simulink model "System_Design_Quadrocopter"  (Simulink 7.5)
settings: Solver=ode45  StartTime=0.0  StopTime=30  RelTol=1e-3
values from neighbouring files (symbols this model uses):
  phi0 = 0.15    [Quadrocopter_control_Driver.m]    (also in calc_stability.m = 0)
  r_phi0 = 0    [Quadrocopter_control_Driver.m]    (also in calc_stability.m)
  r_psi0 = 0    [Quadrocopter_control_Driver.m]    (also in calc_stability.m)
  r_theta0 = 0    [Quadrocopter_control_Driver.m]    (also in calc_stability.m)
  theta0 = 0.15    [Quadrocopter_control_Driver.m]    (also in calc_stability.m = 0)
  Ts = 0.01    [Reglerauslegung.m]    (also in Test_Reglerauslegung.m)
undefined symbols (not defined in the file or in its folder): bodyCtrl_phiCtrl_KD, bodyCtrl_phiCtrl_KI, bodyCtrl_phiCtrl_KP, bodyCtrl_rphiCtrl_KD, bodyCtrl_rphiCtrl_KI, bodyCtrl_rphiCtrl_KP, bodyCtrl_rpsiCtrl_KD, bodyCtrl_rpsiCtrl_KI, bodyCtrl_rpsiCtrl_KP, bodyCtrl_rthetaCtrl_KD, bodyCtrl_rthetaCtrl_KI, bodyCtrl_rthetaCtrl_KP, bodyCtrl_thetaCtrl_KD, bodyCtrl_thetaCtrl_KI, bodyCtrl_thetaCtrl_KP, boom, f1, f2, f3, f4, f5, g, I_x, I_y, I_z, m, positionCtrl_rpsiCtrl_KD, positionCtrl_rpsiCtrl_KI, positionCtrl_rpsiCtrl_KP, sigbuilder_block, speed, thrust, Ts_Opt
libraries: simulink x39, dspobslib x4, Copter_Library x3, Control_lib x1, sdolib x1
(part 3 of 4)

== system System_Design_Quadrocopter/Quadrocopter/Remote Control/Remote_Control_3d_mouse ==
  note: phi(roll)
      | theta(pitch)
      | rpsi(yaw rate)
      | T(thrust)
  Enable : EnablePort  PropagateVarSize=During execution
  Add : Sum
  Add1 : Sum
  Add2 : Sum
  Constant1 : Constant  Value=128
  Constant2 : Constant  Value=128
  Constant3 : Constant  Value=400
  Constant4 : Constant  Value=128
  Demux : Demux  Outputs=3
  Demux1 : Demux  Outputs=3
  Gain1 : Gain
  Mux2 : Mux
  Saturation : Saturate  UpperLimit=255  LowerLimit=0
  Saturation1 : Saturate  UpperLimit=255  LowerLimit=0
  Saturation2 : Saturate  UpperLimit=255  LowerLimit=0
  Saturation3 : Saturate  UpperLimit=inf  LowerLimit=0
  Space Mouse Input : S-Function  AncestorBlock=vrlib/Space Mouse Input  FunctionName=spacemouse  Parameters=Port, OutputType, InitialPosition, InitialRotation, PositionSensitivity, RotationSensitivity, Dominant, NormalizeAngle, DisableTranslation, DisableRotation, PositionLow, PositionUp, EnableLimit  EnableBusSupport=off  mask(Space Mouse Input){Port=USB1, OutputType=Speed, Dominant=off, DisableTranslation=off, DisableRotation=off, NormalizeAngle=off, EnableLimit=on, PositionSensitivity=0.5, RotationSensitivity=2, InitialPosition=[0 0 0], InitialRotation=[0 0 0], PositionLow=[0 0 0], PositionUp=[255 255 255]}
      mask prompts: OutputType "Output type:"; Dominant "Dominant mode"; DisableTranslation "Disable position movement"; DisableRotation "Disable rotation movement"; NormalizeAngle "Normalize output angle"; EnableLimit "Limit position"; PositionSensitivity "Position sensitivity:"; RotationSensitivity "Rotation sensitivity:"; InitialPosition "Initial position:"; InitialRotation "Initial rotation:"; PositionLow "Lower position limit:"; PositionUp "Upper position limit:"
      mask help: Space Mouse input device driver.
      mask Help: helpview(fullfile(docroot, 'toolbox', 'sl3d', 'sl3d.map'), 'vr_magellanspacemouse');
      mask StyleString: popup(COM1|COM2|COM3|COM4|USB1|USB2|USB3|USB4|USB),popup(Speed|Position|Viewpoint coordinates),checkbox,checkbox,checkbox,checkbox,checkbox,edit,edit,edit,edit,edit,edit
      mask CallbackString: spacemousemask|spacemousemask|||||spacemousemask||||||
      mask Display:
      | image(imread('spacemouseicon.png'))
      | port_label('output', 1, 'Translation')
      | port_label('output', 2, 'Rotation')
      | port_label('output', 3, 'Buttons')
  Out1 : Outport
  wires:
  Demux/1 -> Add2/1  "phi_set"
  Constant4/1 -> Add2/2
  Demux/3 -> Add1/1  "theta_set"
  Constant2/1 -> Add1/2
  Add/1 -> Saturation2/1
  Demux1/2 -> Add/1  "psi_set"
  Constant1/1 -> Add/2
  Space Mouse Input/2 -> Demux1/1  "[Kippen, Rollen, Drehen]"
  Space Mouse Input/1 -> Demux/1  "[Trans_X, Trans_Z, Trans_Y]"
  Gain1/1 -> Mux2/4  "thrust"
  Mux2/1 -> Out1/1
  Add2/1 -> Saturation/1
  Add1/1 -> Saturation1/1
  Saturation1/1 -> Mux2/2
  Saturation2/1 -> Mux2/3
  Saturation/1 -> Mux2/1
  Saturation3/1 -> Gain1/1
  Demux/2 -> Saturation3/1  "Zoom"

== system System_Design_Quadrocopter/Quadrocopter/Remote Control/Square_path_stimuli ==
  note: phi(roll)
      | theta(pitch)
      | rpsi(yaw rate)
      | T(thrust)
  Add{,1..3} (4 alike) : Sum  OutDataType=fixdt(1, 16)  OutScaling=2^-10
  Constant{,1..3} (4 alike) : Constant  Value=128  OutDataType=fixdt(1, 16)  OutScaling=2^0
  Gain : Gain  ParameterDataType=fixdt(1, 16)  ParameterScaling=2^0  OutDataType=fixdt(1, 16)  OutScaling=2^0
  Mux1 : Mux
  Signal Builder : Subsystem  Tag=STV Subsys  LoadFcn=sigbuilder_block('load');  StartFcn=sigbuilder_block('start');  StopFcn=sigbuilder_block('stop');  ClipboardFcn=sigbuilder_block('clipboard');  mask(Sigbuilder block){}
      mask help: Create and generate interchangeable groups of signals whose waveforms are piecewise linear.
      mask init:
      | if ~strcmp(get_param(bdroot(gcbh),'SimulationStatus'),'stopped') tuvar = sigbuilder_block('maskInit'); end
      settings: CopyFcn=sigbuilder_block('copy');  DeleteFcn=sigbuilder_block('delete');  ModelCloseFcn=sigbuilder_block('modelClose');  PreSaveFcn=sigbuilder_block('preSave');  NameChangeFcn=sigbuilder_block('namechange');  OpenFcn=sigbuilder_block('open',[437.25 199.5 550.5 399.75 ]);  CloseFcn=sigbuilder_block('close');
      mask Display: plot(0,0,100,100,[10,10,40,40,10],[80,20,20,80,80],[40,10],[50,50], [40,27,10],[65,72,56],[40,25,25,10],[28,28,43,43]);
  Subsystem1 : Subsystem  mask{Gain_=-40}
      mask prompts: Gain_ "Gain"
  Subsystem2 : Subsystem  mask{Gain_=-40}
      mask prompts: Gain_ "Gain"
  Subsystem3 : Subsystem  mask{Gain_=40}
      mask prompts: Gain_ "Gain"
  Subsystem4 : Subsystem  mask{Gain_=40}
      mask prompts: Gain_ "Gain"
  Out : Outport  OutDataType=fixdt(1, 16)  OutScaling=2^0
  wires:
  Mux1/1 -> Out/1
  Constant2/1 -> Mux1/3  "rpsi_set"
  Constant/1 -> Gain/1
  Gain/1 -> Mux1/4  "thrust"
  Subsystem3/1(Out1) -> Add1/1
  Subsystem1/1(Out1) -> Add1/2
  Constant3/1 -> Add/1
  Add/1 -> Mux1/1
  Subsystem4/1(Out1) -> Add2/1
  Subsystem2/1(Out1) -> Add2/2
  Add2/1 -> Add/2
  Add1/1 -> Add3/2
  Add3/1 -> Mux1/2
  Constant1/1 -> Add3/1
  Signal Builder/1(Signal 1) -> Subsystem4/1(In1)
  Signal Builder/2(Signal 2) -> Subsystem3/1(In1)
  Signal Builder/3(Signal 3) -> Subsystem2/1(In1)
  Signal Builder/4(Signal 4) -> Subsystem1/1(In1)

== system System_Design_Quadrocopter/Quadrocopter/Remote Control/Step_Stimuli ==
  note: phi(roll)
      | theta(pitch)
      | rpsi(yaw rate)
      | T(thrust)
  Add : Sum  OutDataType=fixdt(1, 16)  OutScaling=2^-10
  Add1 : Sum  OutDataType=fixdt(1, 16)  OutScaling=2^-10
  Add2 : Sum  OutDataType=fixdt(1, 16)  OutScaling=2^-10
  Constant{,1,3..4} (4 alike) : Constant  Value=128  OutDataType=fixdt(1, 16)  OutScaling=2^0
  Gain : Gain  ParameterDataType=fixdt(1, 16)  ParameterScaling=2^0  OutDataType=fixdt(1, 16)  OutScaling=2^0
  Mux1 : Mux
  Step_phi : Step  Time=[5]  After=[-128]  SampleTime=0
  Step_psi : Step  Time=[0]  After=[0]  SampleTime=0
  Step_theta : Step  Time=[5]  After=[0]  SampleTime=0
  Out : Outport  OutDataType=fixdt(1, 16)  OutScaling=2^0
  wires:
  Mux1/1 -> Out/1
  Constant/1 -> Gain/1
  Gain/1 -> Mux1/4  "thrust"
  Constant3/1 -> Add/2
  Add/1 -> Mux1/1
  Step_theta/1 -> Add1/1
  Constant4/1 -> Add1/2
  Add1/1 -> Mux1/2
  Step_psi/1 -> Add2/1
  Constant1/1 -> Add2/2
  Add2/1 -> Mux1/3
  Step_phi/1 -> Add/1

== system System_Design_Quadrocopter/Quadrocopter/SDO/captrPsi ==
  In2 : Inport
  Terminator : Terminator
  To File : ToFile  Filename=SDO_51.mat
  cntr : Constant  Value=<binary blob, 1398102 chars, not shown>  OutDataType=fixdt(1, 16)  OutScaling=2^0
  wires:
  In2/1 -> To File/1
  cntr/1 -> Terminator/1

== system System_Design_Quadrocopter/Quadrocopter/Sensors/Optical System ==
  note: %opt_sensor_record
      | %[
      | 1:Opt_Var_Trans
      | 2:Opt_Var_ST_Trans
      | 3:Opt_Limit_Trans
      | 4:Opt_Ori_SG_Trans
      | 5:Opt_Var_Rot
      | 6:Opt_Var_ST_Rot
      | 7:Opt_Limit_Rot
      | 8:Opt_Ori_SG_Rot
      | 9:Opt_Delay_Global
      | 10:Opt_ST_Global]
  IdealSigs : Inport
  Demux1 : Demux  Outputs=3
  Mux1 : Mux  Inputs=3
  Rotation rpsi : Subsystem  mask{Opt_Var=Opt_Sens_Rec(5), Opt_Var_ST=Opt_Sens_Rec(6), Opt_Limit=Opt_Sens_Rec(7), Opt_Delay=Opt_Sens_Rec(9), Opt_ST=Opt_Sens_Rec(10), Opt_Ori_SG=Opt_Sens_Rec(8)}
      mask prompts: Opt_Var "Variance"; Opt_Var_ST "Sample Time of Variance"; Opt_Limit "Limitation [m/s]"; Opt_Delay "Delay"; Opt_ST "Sample Time (1/Frame Rate)"; Opt_Ori_SG "Original Signal Gain"
  Scope : Scope
      settings: YMin=-0.5  YMax=7  SaveName=ScopeData23
  Translation VX : Subsystem  mask{Opt_Var=Opt_Sens_Rec(1), Opt_Var_ST=Opt_Sens_Rec(2), Opt_Limit=Opt_Sens_Rec(3), Opt_Delay=Opt_Sens_Rec(9), Opt_ST=Opt_Sens_Rec(10), Opt_Ori_SG=Opt_Sens_Rec(4)}
      mask prompts: Opt_Var "Variance"; Opt_Var_ST "Sample Time of Variance"; Opt_Limit "Limitation [m/s]"; Opt_Delay "Delay"; Opt_ST "Sample Time (1/Frame Rate)"; Opt_Ori_SG "Original Signal Gain"
  Translation VY : Subsystem  mask{Opt_Var=Opt_Sens_Rec(1), Opt_Var_ST=Opt_Sens_Rec(2), Opt_Limit=Opt_Sens_Rec(3), Opt_Delay=Opt_Sens_Rec(9), Opt_ST=Opt_Sens_Rec(10), Opt_Ori_SG=Opt_Sens_Rec(4)}
      mask prompts: Opt_Var "Variance"; Opt_Var_ST "Sample Time of Variance"; Opt_Limit "Limitation [m/s]"; Opt_Delay "Delay"; Opt_ST "Sample Time (1/Frame Rate)"; Opt_Ori_SG "Original Signal Gain"
  SensorSigs : Outport
  wires:
  Demux1/1 -> Translation VX/1(IdealSig)
  Demux1/2 -> Translation VY/1(IdealSig)
  Demux1/3 -> Rotation rpsi/1(IdealSig)
  Translation VX/1(OptSig) -> Mux1/1
  Translation VY/1(OptSig) -> Mux1/2
  Rotation rpsi/1(OptSig) -> Mux1/3
  IdealSigs/1 -> Demux1/1
  Mux1/1 -> SensorSigs/1, Scope/1

== system System_Design_Quadrocopter/Quadrocopter/Sensors/acc_ax_sensor ==
  note: inverted work like the real copter
  ax : Inport
  Enable Noise : Inport  Port=2
  Gain17 : Gain  Gain=g
  Gain30 : Gain  Gain=-340/g
  Quantizer4 : Quantizer  QuantizationInterval=g/340  SampleTime=Ts
  Saturation : Saturate  UpperLimit=6*g  LowerLimit=-6*g  OutDataType=fixdt(1, 16)  OutScaling=2^0
  Sensor Noise : Subsystem
  Sum15 : Sum
  Trigonometric Function : Trigonometry
  ax_sens : Outport
  wires:
  Sensor Noise/1(Noise) -> Sum15/1
  Sum15/1 -> Saturation/1
  Gain17/1 -> Sum15/2
  Quantizer4/1 -> Gain30/1
  Gain30/1 -> ax_sens/1
  Enable Noise/1 -> Sensor Noise/Enable
  Saturation/1 -> Quantizer4/1
  ax/1 -> Trigonometric Function/1
  Trigonometric Function/1 -> Gain17/1

== system System_Design_Quadrocopter/Quadrocopter/Sensors/acc_ay_sensor ==
  note: inverted like in the real copter
  phi : Inport
  Enable Noise : Inport  Port=2
  Gain19 : Gain  Gain=-340/g
  Gain22 : Gain  Gain=g
  Quantizer3 : Quantizer  QuantizationInterval=g/340  SampleTime=Ts
  Saturation : Saturate  UpperLimit=6*g  LowerLimit=-6*g  OutDataType=fixdt(1, 16)  OutScaling=2^0
  Sensor Noise : Subsystem
  Sum12 : Sum
  Trigonometric Function : Trigonometry
  ay_sens : Outport
  wires:
  Sum12/1 -> Saturation/1
  Quantizer3/1 -> Gain19/1
  phi/1 -> Trigonometric Function/1
  Gain19/1 -> ay_sens/1
  Enable Noise/1 -> Sensor Noise/Enable
  Sensor Noise/1(Noise) -> Sum12/1
  Saturation/1 -> Quantizer3/1
  Gain22/1 -> Sum12/2
  Trigonometric Function/1 -> Gain22/1

== system System_Design_Quadrocopter/Quadrocopter/Sensors/rate_phi_sensor ==
  note: Sensor adds noise and Samples and quantize the Signal. In combination with the gain a integer value is generated
      | like the Sensor is read from the ADC registers.
  r_phi : Inport
  Enable Noise : Inport  Port=2
  Gain20 : Gain  Gain=1/0.00938349
  Offset : Constant  Value=505
  Quantizer : Quantizer  QuantizationInterval=0.00938349  SampleTime=Ts
  Sensor Noise : Subsystem
  Sum : Sum  Inputs=++|
  Sum14 : Sum
  r_phi_sens : Outport
  wires:
  Sum14/1 -> Quantizer/1
  Quantizer/1 -> Gain20/1
  r_phi/1 -> Sum14/2
  Gain20/1 -> Sum/2
  Offset/1 -> Sum/1
  Sum/1 -> r_phi_sens/1
  Enable Noise/1 -> Sensor Noise/Enable
  Sensor Noise/1(Noise) -> Sum14/1

== system System_Design_Quadrocopter/Quadrocopter/Sensors/rate_psi_sensor ==
  note: Gyroscope / Acceleration Sensor
  sig_in : Inport
  enable_noise_in : Inport  Port=2
  Gain : Gain  Gain=-1/0.00938349
  Offset : Constant  Value=505
  Quantizer : Quantizer  QuantizationInterval=0.00938349  SampleTime=Ts
  Sensor Noise : Subsystem
  Sum : Sum  Inputs=++|
  Sum13 : Sum
  sens_out : Outport
  wires:
  Sensor Noise/1(Noise) -> Sum13/1
  sig_in/1 -> Sum13/2
  Offset/1 -> Sum/1
  Gain/1 -> Sum/2
  Sum/1 -> sens_out/1
  enable_noise_in/1 -> Sensor Noise/Enable
  Quantizer/1 -> Gain/1
  Sum13/1 -> Quantizer/1

== system System_Design_Quadrocopter/Quadrocopter/Sensors/rate_theta_sensor ==
  note: inverted to worj like in the real copter
  r_theta : Inport
  Enable Noise : Inport  Port=2
  Gain27 : Gain  Gain=-1/0.00938349
  Offset : Constant  Value=505
  Quantizer1 : Quantizer  QuantizationInterval=0.00938349  SampleTime=Ts
  Sensor Noise : Subsystem
  Sum : Sum  Inputs=++|
  Sum16 : Sum
  r_theta_sens : Outport
  wires:
  Sum16/1 -> Quantizer1/1
  Quantizer1/1 -> Gain27/1
  r_theta/1 -> Sum16/2
  Offset/1 -> Sum/1
  Gain27/1 -> Sum/2
  Sum/1 -> r_theta_sens/1
  Enable Noise/1 -> Sensor Noise/Enable
  Sensor Noise/1(Noise) -> Sum16/1

== system System_Design_Quadrocopter/Quadrocopter/Control/PID_Control_IMU Rot Trans (OC)/Control Hovering Mode ==
  vx_opt : Inport  OutDataType=fixdt(1, 16)  OutScaling=2^0
  theta_hm_set : Inport  Port=2  OutDataType=fixdt(1, 16)  OutScaling=2^0
  phi_hm_set : Inport  Port=3  OutDataType=fixdt(1, 16)  OutScaling=2^0
  vy_opt : Inport  Port=4  OutDataType=fixdt(1, 16)  OutScaling=2^0
  rpsi_opt : Inport  Port=5  OutDataType=fixdt(1, 16)  OutScaling=2^0
  rpsi_hm_set : Inport  Port=6  OutDataType=fixdt(1, 16)  OutScaling=2^0
  Enable : EnablePort  ZeroCross=off
  Gain : Gain  ParameterDataType=fixdt(1, 16)  ParameterScaling=2^0  OutDataType=fixdt(1, 16)  OutScaling=2^0
  Gain1 : Gain  ParameterDataType=fixdt(1, 16)  ParameterScaling=2^0  OutDataType=fixdt(1, 16)  OutScaling=2^0
  Gain6 : Gain  ParameterDataType=fixdt(1, 16)  ParameterScaling=2^0  OutDataType=fixdt(1, 16)  OutScaling=2^0
  PID rPhi OPT : simulink/Continuous/PID Controller  DialogController=pidpack.PIDConfig.pidDDGCreate  DialogControllerArgs=DataTag6  SystemSampleTime=-1  Controller=PID  TimeDomain=Discrete-time  SampleTime=Ts_Opt  IntegratorMethod=Forward Euler  FilterMethod=Forward Euler  Form=Ideal  P=10  I=0.5  D=0  N=2  InitialConditionSource=internal  InitialConditionForIntegrator=0  InitialConditionForFilter=0  ExternalReset=none  ZeroCross=off  LimitOutput=off  UpperSaturationLimit=inf  LowerSaturationLimit=-inf  LinearizeAsGain=off  AntiWindupMode=clamping  Kb=1  TrackingMode=off  Kt=1  PParamMin=[]  PParamMax=[]  IParamMin=[]  IParamMax=[]  DParamMin=[]  DParamMax=[]  NParamMin=[]  NParamMax=[]  KbParamMin=[]  KbParamMax=[]  KtParamMin=[]  KtParamMax=[]  POutMin=[]  POutMax=[]  IOutMin=[]  IOutMax=[]  DOutMin=[]  DOutMax=[]  NOutMin=[]  NOutMax=[]  KbOutMin=[]  KbOutMax=[]  KtOutMin=[]  KtOutMax=[]  IntegratorOutMin=[]  IntegratorOutMax=[]  FilterOutMin=[]  FilterOutMax=[]  SumOutMin=[]  SumOutMax=[]  SumI1OutMin=[]  SumI1OutMax=[]  SumI2OutMin=[]  SumI2OutMax=[]  SumI3OutMin=[]  SumI3OutMax=[]  SumDOutMin=[]  SumDOutMax=[]  SaturationOutMin=[]  SaturationOutMax=[]  IntegratorContinuousStateAttributes=''  IntegratorStateMustResolveToSignalObject=off  IntegratorRTWStateStorageClass=Auto  FilterContinuousStateAttributes=''  FilterStateMustResolveToSignalObject=off  FilterRTWStateStorageClass=Auto
  PID rPsi OPT : simulink/Continuous/PID Controller  DialogController=pidpack.PIDConfig.pidDDGCreate  DialogControllerArgs=DataTag7  SystemSampleTime=-1  Controller=PID  TimeDomain=Discrete-time  SampleTime=Ts_Opt  IntegratorMethod=Forward Euler  FilterMethod=Forward Euler  Form=Ideal  P=10  I=0.5  D=0  N=0  InitialConditionSource=internal  InitialConditionForIntegrator=0  InitialConditionForFilter=0  ExternalReset=none  ZeroCross=off  LimitOutput=off  UpperSaturationLimit=inf  LowerSaturationLimit=-inf  LinearizeAsGain=off  AntiWindupMode=clamping  Kb=1  TrackingMode=off  Kt=1  PParamMin=[]  PParamMax=[]  IParamMin=[]  IParamMax=[]  DParamMin=[]  DParamMax=[]  NParamMin=[]  NParamMax=[]  KbParamMin=[]  KbParamMax=[]  KtParamMin=[]  KtParamMax=[]  POutMin=[]  POutMax=[]  IOutMin=[]  IOutMax=[]  DOutMin=[]  DOutMax=[]  NOutMin=[]  NOutMax=[]  KbOutMin=[]  KbOutMax=[]  KtOutMin=[]  KtOutMax=[]  IntegratorOutMin=[]  IntegratorOutMax=[]  FilterOutMin=[]  FilterOutMax=[]  SumOutMin=[]  SumOutMax=[]  SumI1OutMin=[]  SumI1OutMax=[]  SumI2OutMin=[]  SumI2OutMax=[]  SumI3OutMin=[]  SumI3OutMax=[]  SumDOutMin=[]  SumDOutMax=[]  SaturationOutMin=[]  SaturationOutMax=[]  IntegratorContinuousStateAttributes=''  IntegratorStateMustResolveToSignalObject=off  IntegratorRTWStateStorageClass=Auto  FilterContinuousStateAttributes=''  FilterStateMustResolveToSignalObject=off  FilterRTWStateStorageClass=Auto
  PID rTheta OPT : simulink/Continuous/PID Controller  DialogController=pidpack.PIDConfig.pidDDGCreate  DialogControllerArgs=DataTag8  SystemSampleTime=-1  Controller=PID  TimeDomain=Discrete-time  SampleTime=Ts_Opt  IntegratorMethod=Forward Euler  FilterMethod=Forward Euler  Form=Ideal  P=10  I=0.5  D=0  N=0  InitialConditionSource=internal  InitialConditionForIntegrator=0  InitialConditionForFilter=0  ExternalReset=none  ZeroCross=off  LimitOutput=off  UpperSaturationLimit=inf  LowerSaturationLimit=-inf  LinearizeAsGain=off  AntiWindupMode=clamping  Kb=1  TrackingMode=off  Kt=1  PParamMin=[]  PParamMax=[]  IParamMin=[]  IParamMax=[]  DParamMin=[]  DParamMax=[]  NParamMin=[]  NParamMax=[]  KbParamMin=[]  KbParamMax=[]  KtParamMin=[]  KtParamMax=[]  POutMin=[]  POutMax=[]  IOutMin=[]  IOutMax=[]  DOutMin=[]  DOutMax=[]  NOutMin=[]  NOutMax=[]  KbOutMin=[]  KbOutMax=[]  KtOutMin=[]  KtOutMax=[]  IntegratorOutMin=[]  IntegratorOutMax=[]  FilterOutMin=[]  FilterOutMax=[]  SumOutMin=[]  SumOutMax=[]  SumI1OutMin=[]  SumI1OutMax=[]  SumI2OutMin=[]  SumI2OutMax=[]  SumI3OutMin=[]  SumI3OutMax=[]  SumDOutMin=[]  SumDOutMax=[]  SaturationOutMin=[]  SaturationOutMax=[]  IntegratorContinuousStateAttributes=''  IntegratorStateMustResolveToSignalObject=off  IntegratorRTWStateStorageClass=Auto  FilterContinuousStateAttributes=''  FilterStateMustResolveToSignalObject=off  FilterRTWStateStorageClass=Auto
  Sum1 : Sum  Inputs=|+-  OutDataType=fixdt(1, 16)  OutScaling=2^0
  Sum16 : Sum  Inputs=|+-  OutDataType=fixdt(1, 16)  OutScaling=2^0
  Sum2 : Sum  Inputs=|+-  OutDataType=fixdt(1, 16)  OutScaling=2^0
  m_theta : Outport  OutDataType=fixdt(1, 16)  OutScaling=2^0
  m_phi : Outport  Port=2  OutDataType=fixdt(1, 16)  OutScaling=2^0
  m_psi : Outport  Port=3  OutDataType=fixdt(1, 16)  OutScaling=2^0
  wires:
  Gain6/1 -> Sum16/2
  Sum16/1 -> PID rTheta OPT/1  "e_theta_hm"
  theta_hm_set/1 -> Sum16/1
  Sum2/1 -> PID rPhi OPT/1  "e_phi_hm"
  PID rPhi OPT/1 -> m_phi/1
  Gain1/1 -> Sum2/2
  vx_opt/1 -> Gain6/1
  PID rTheta OPT/1 -> m_theta/1
  phi_hm_set/1 -> Sum2/1
  rpsi_hm_set/1 -> Sum1/1
  PID rPsi OPT/1 -> Gain/1
  vy_opt/1 -> Gain1/1
  Sum1/1 -> PID rPsi OPT/1
  rpsi_opt/1 -> Sum1/2
  Gain/1 -> m_psi/1

== system System_Design_Quadrocopter/Quadrocopter/Control/PID_Control_IMU Rot Trans (OC) EMP/Control Hovering Mode ==
  vx_opt : Inport  OutDataType=fixdt(1, 16)  OutScaling=2^0
  theta_hm_set : Inport  Port=2  OutDataType=fixdt(1, 16)  OutScaling=2^0
  phi_hm_set : Inport  Port=3  OutDataType=fixdt(1, 16)  OutScaling=2^0
  vy_opt : Inport  Port=4  OutDataType=fixdt(1, 16)  OutScaling=2^0
  rpsi_opt : Inport  Port=5  OutDataType=fixdt(1, 16)  OutScaling=2^0
  rpsi_hm_set : Inport  Port=6  OutDataType=fixdt(1, 16)  OutScaling=2^0
  Enable : EnablePort  ZeroCross=off
  Gain : Gain  ParameterDataType=fixdt(1, 16)  ParameterScaling=2^0  OutDataType=fixdt(1, 16)  OutScaling=2^0
  Gain1 : Gain  ParameterDataType=fixdt(1, 16)  ParameterScaling=2^0  OutDataType=fixdt(1, 16)  OutScaling=2^0
  Gain6 : Gain  ParameterDataType=fixdt(1, 16)  ParameterScaling=2^0  OutDataType=fixdt(1, 16)  OutScaling=2^0
  PID rPhi OPT : simulink/Continuous/PID Controller  DialogController=pidpack.PIDConfig.pidDDGCreate  DialogControllerArgs=DataTag14  SystemSampleTime=-1  Controller=PID  TimeDomain=Discrete-time  SampleTime=Ts_Opt  IntegratorMethod=Forward Euler  FilterMethod=Forward Euler  Form=Ideal  P=10  I=0.5  D=0  N=2  InitialConditionSource=internal  InitialConditionForIntegrator=0  InitialConditionForFilter=0  ExternalReset=none  ZeroCross=off  LimitOutput=off  UpperSaturationLimit=inf  LowerSaturationLimit=-inf  LinearizeAsGain=off  AntiWindupMode=clamping  Kb=1  TrackingMode=off  Kt=1  PParamMin=[]  PParamMax=[]  IParamMin=[]  IParamMax=[]  DParamMin=[]  DParamMax=[]  NParamMin=[]  NParamMax=[]  KbParamMin=[]  KbParamMax=[]  KtParamMin=[]  KtParamMax=[]  POutMin=[]  POutMax=[]  IOutMin=[]  IOutMax=[]  DOutMin=[]  DOutMax=[]  NOutMin=[]  NOutMax=[]  KbOutMin=[]  KbOutMax=[]  KtOutMin=[]  KtOutMax=[]  IntegratorOutMin=[]  IntegratorOutMax=[]  FilterOutMin=[]  FilterOutMax=[]  SumOutMin=[]  SumOutMax=[]  SumI1OutMin=[]  SumI1OutMax=[]  SumI2OutMin=[]  SumI2OutMax=[]  SumI3OutMin=[]  SumI3OutMax=[]  SumDOutMin=[]  SumDOutMax=[]  SaturationOutMin=[]  SaturationOutMax=[]  IntegratorContinuousStateAttributes=''  IntegratorStateMustResolveToSignalObject=off  IntegratorRTWStateStorageClass=Auto  FilterContinuousStateAttributes=''  FilterStateMustResolveToSignalObject=off  FilterRTWStateStorageClass=Auto
  PID rPsi OPT : simulink/Continuous/PID Controller  DialogController=pidpack.PIDConfig.pidDDGCreate  DialogControllerArgs=DataTag15  SystemSampleTime=-1  Controller=PID  TimeDomain=Discrete-time  SampleTime=Ts_Opt  IntegratorMethod=Forward Euler  FilterMethod=Forward Euler  Form=Ideal  P=positionCtrl_rpsiCtrl_KP  I=positionCtrl_rpsiCtrl_KI  D=positionCtrl_rpsiCtrl_KD  N=0  InitialConditionSource=internal  InitialConditionForIntegrator=0  InitialConditionForFilter=0  ExternalReset=none  ZeroCross=off  LimitOutput=off  UpperSaturationLimit=inf  LowerSaturationLimit=-inf  LinearizeAsGain=off  AntiWindupMode=clamping  Kb=1  TrackingMode=off  Kt=1  PParamMin=[]  PParamMax=[]  IParamMin=[]  IParamMax=[]  DParamMin=[]  DParamMax=[]  NParamMin=[]  NParamMax=[]  KbParamMin=[]  KbParamMax=[]  KtParamMin=[]  KtParamMax=[]  POutMin=[]  POutMax=[]  IOutMin=[]  IOutMax=[]  DOutMin=[]  DOutMax=[]  NOutMin=[]  NOutMax=[]  KbOutMin=[]  KbOutMax=[]  KtOutMin=[]  KtOutMax=[]  IntegratorOutMin=[]  IntegratorOutMax=[]  FilterOutMin=[]  FilterOutMax=[]  SumOutMin=[]  SumOutMax=[]  SumI1OutMin=[]  SumI1OutMax=[]  SumI2OutMin=[]  SumI2OutMax=[]  SumI3OutMin=[]  SumI3OutMax=[]  SumDOutMin=[]  SumDOutMax=[]  SaturationOutMin=[]  SaturationOutMax=[]  IntegratorContinuousStateAttributes=''  IntegratorStateMustResolveToSignalObject=off  IntegratorRTWStateStorageClass=Auto  FilterContinuousStateAttributes=''  FilterStateMustResolveToSignalObject=off  FilterRTWStateStorageClass=Auto
  PID rTheta OPT : simulink/Continuous/PID Controller  DialogController=pidpack.PIDConfig.pidDDGCreate  DialogControllerArgs=DataTag16  SystemSampleTime=-1  Controller=PID  TimeDomain=Discrete-time  SampleTime=Ts_Opt  IntegratorMethod=Forward Euler  FilterMethod=Forward Euler  Form=Ideal  P=10  I=0.5  D=0  N=0  InitialConditionSource=internal  InitialConditionForIntegrator=0  InitialConditionForFilter=0  ExternalReset=none  ZeroCross=off  LimitOutput=off  UpperSaturationLimit=inf  LowerSaturationLimit=-inf  LinearizeAsGain=off  AntiWindupMode=clamping  Kb=1  TrackingMode=off  Kt=1  PParamMin=[]  PParamMax=[]  IParamMin=[]  IParamMax=[]  DParamMin=[]  DParamMax=[]  NParamMin=[]  NParamMax=[]  KbParamMin=[]  KbParamMax=[]  KtParamMin=[]  KtParamMax=[]  POutMin=[]  POutMax=[]  IOutMin=[]  IOutMax=[]  DOutMin=[]  DOutMax=[]  NOutMin=[]  NOutMax=[]  KbOutMin=[]  KbOutMax=[]  KtOutMin=[]  KtOutMax=[]  IntegratorOutMin=[]  IntegratorOutMax=[]  FilterOutMin=[]  FilterOutMax=[]  SumOutMin=[]  SumOutMax=[]  SumI1OutMin=[]  SumI1OutMax=[]  SumI2OutMin=[]  SumI2OutMax=[]  SumI3OutMin=[]  SumI3OutMax=[]  SumDOutMin=[]  SumDOutMax=[]  SaturationOutMin=[]  SaturationOutMax=[]  IntegratorContinuousStateAttributes=''  IntegratorStateMustResolveToSignalObject=off  IntegratorRTWStateStorageClass=Auto  FilterContinuousStateAttributes=''  FilterStateMustResolveToSignalObject=off  FilterRTWStateStorageClass=Auto
  Sum1 : Sum  Inputs=|+-  OutDataType=fixdt(1, 16)  OutScaling=2^0
  Sum16 : Sum  Inputs=|+-  OutDataType=fixdt(1, 16)  OutScaling=2^0
  Sum2 : Sum  Inputs=|+-  OutDataType=fixdt(1, 16)  OutScaling=2^0
  m_theta : Outport  OutDataType=fixdt(1, 16)  OutScaling=2^0
  m_phi : Outport  Port=2  OutDataType=fixdt(1, 16)  OutScaling=2^0
  m_psi : Outport  Port=3  OutDataType=fixdt(1, 16)  OutScaling=2^0
  wires:
  Gain6/1 -> Sum16/2
  Sum16/1 -> PID rTheta OPT/1  "e_theta_hm"
  theta_hm_set/1 -> Sum16/1
  Sum2/1 -> PID rPhi OPT/1  "e_phi_hm"
  PID rPhi OPT/1 -> m_phi/1
  Gain1/1 -> Sum2/2
  vx_opt/1 -> Gain6/1
  PID rTheta OPT/1 -> m_theta/1
  phi_hm_set/1 -> Sum2/1
  rpsi_hm_set/1 -> Sum1/1
  PID rPsi OPT/1 -> Gain/1
  vy_opt/1 -> Gain1/1
  Sum1/1 -> PID rPsi OPT/1
  rpsi_opt/1 -> Sum1/2
  Gain/1 -> m_psi/1

== system System_Design_Quadrocopter/Quadrocopter/Control/PID_Control_IMU only Trans (OC)/Control Hovering Mode ==
  vx_opt : Inport  OutDataType=fixdt(1, 16)  OutScaling=2^0
  theta_hm_set : Inport  Port=2  OutDataType=fixdt(1, 16)  OutScaling=2^0
  phi_hm_set : Inport  Port=3  OutDataType=fixdt(1, 16)  OutScaling=2^0
  vy_opt : Inport  Port=4  OutDataType=fixdt(1, 16)  OutScaling=2^0
  rpsi_opt : Inport  Port=5  OutDataType=fixdt(1, 16)  OutScaling=2^0
  rpsi_hm_set : Inport  Port=6  OutDataType=fixdt(1, 16)  OutScaling=2^0
  Enable : EnablePort  ZeroCross=off
  Gain : Gain  ParameterDataType=fixdt(1, 16)  ParameterScaling=2^0  OutDataType=fixdt(1, 16)  OutScaling=2^0
  Gain1 : Gain  ParameterDataType=fixdt(1, 16)  ParameterScaling=2^0  OutDataType=fixdt(1, 16)  OutScaling=2^0
  Gain6 : Gain  ParameterDataType=fixdt(1, 16)  ParameterScaling=2^0  OutDataType=fixdt(1, 16)  OutScaling=2^0
  PID rPhi OPT : simulink/Continuous/PID Controller  DialogController=pidpack.PIDConfig.pidDDGCreate  DialogControllerArgs=DataTag22  SystemSampleTime=-1  Controller=PID  TimeDomain=Discrete-time  SampleTime=Ts_Opt  IntegratorMethod=Forward Euler  FilterMethod=Forward Euler  Form=Ideal  P=10  I=0.5  D=0  N=2  InitialConditionSource=internal  InitialConditionForIntegrator=0  InitialConditionForFilter=0  ExternalReset=none  ZeroCross=off  LimitOutput=off  UpperSaturationLimit=inf  LowerSaturationLimit=-inf  LinearizeAsGain=off  AntiWindupMode=clamping  Kb=1  TrackingMode=off  Kt=1  PParamMin=[]  PParamMax=[]  IParamMin=[]  IParamMax=[]  DParamMin=[]  DParamMax=[]  NParamMin=[]  NParamMax=[]  KbParamMin=[]  KbParamMax=[]  KtParamMin=[]  KtParamMax=[]  POutMin=[]  POutMax=[]  IOutMin=[]  IOutMax=[]  DOutMin=[]  DOutMax=[]  NOutMin=[]  NOutMax=[]  KbOutMin=[]  KbOutMax=[]  KtOutMin=[]  KtOutMax=[]  IntegratorOutMin=[]  IntegratorOutMax=[]  FilterOutMin=[]  FilterOutMax=[]  SumOutMin=[]  SumOutMax=[]  SumI1OutMin=[]  SumI1OutMax=[]  SumI2OutMin=[]  SumI2OutMax=[]  SumI3OutMin=[]  SumI3OutMax=[]  SumDOutMin=[]  SumDOutMax=[]  SaturationOutMin=[]  SaturationOutMax=[]  IntegratorContinuousStateAttributes=''  IntegratorStateMustResolveToSignalObject=off  IntegratorRTWStateStorageClass=Auto  FilterContinuousStateAttributes=''  FilterStateMustResolveToSignalObject=off  FilterRTWStateStorageClass=Auto
  PID rPsi OPT : simulink/Continuous/PID Controller  DialogController=pidpack.PIDConfig.pidDDGCreate  DialogControllerArgs=DataTag23  SystemSampleTime=-1  Controller=PID  TimeDomain=Discrete-time  SampleTime=Ts_Opt  IntegratorMethod=Forward Euler  FilterMethod=Forward Euler  Form=Ideal  P=10  I=0.5  D=0  N=0  InitialConditionSource=internal  InitialConditionForIntegrator=0  InitialConditionForFilter=0  ExternalReset=none  ZeroCross=off  LimitOutput=off  UpperSaturationLimit=inf  LowerSaturationLimit=-inf  LinearizeAsGain=off  AntiWindupMode=clamping  Kb=1  TrackingMode=off  Kt=1  PParamMin=[]  PParamMax=[]  IParamMin=[]  IParamMax=[]  DParamMin=[]  DParamMax=[]  NParamMin=[]  NParamMax=[]  KbParamMin=[]  KbParamMax=[]  KtParamMin=[]  KtParamMax=[]  POutMin=[]  POutMax=[]  IOutMin=[]  IOutMax=[]  DOutMin=[]  DOutMax=[]  NOutMin=[]  NOutMax=[]  KbOutMin=[]  KbOutMax=[]  KtOutMin=[]  KtOutMax=[]  IntegratorOutMin=[]  IntegratorOutMax=[]  FilterOutMin=[]  FilterOutMax=[]  SumOutMin=[]  SumOutMax=[]  SumI1OutMin=[]  SumI1OutMax=[]  SumI2OutMin=[]  SumI2OutMax=[]  SumI3OutMin=[]  SumI3OutMax=[]  SumDOutMin=[]  SumDOutMax=[]  SaturationOutMin=[]  SaturationOutMax=[]  IntegratorContinuousStateAttributes=''  IntegratorStateMustResolveToSignalObject=off  IntegratorRTWStateStorageClass=Auto  FilterContinuousStateAttributes=''  FilterStateMustResolveToSignalObject=off  FilterRTWStateStorageClass=Auto
  PID rTheta OPT : simulink/Continuous/PID Controller  DialogController=pidpack.PIDConfig.pidDDGCreate  DialogControllerArgs=DataTag24  SystemSampleTime=-1  Controller=PID  TimeDomain=Discrete-time  SampleTime=Ts_Opt  IntegratorMethod=Forward Euler  FilterMethod=Forward Euler  Form=Ideal  P=10  I=0.5  D=0  N=0  InitialConditionSource=internal  InitialConditionForIntegrator=0  InitialConditionForFilter=0  ExternalReset=none  ZeroCross=off  LimitOutput=off  UpperSaturationLimit=inf  LowerSaturationLimit=-inf  LinearizeAsGain=off  AntiWindupMode=clamping  Kb=1  TrackingMode=off  Kt=1  PParamMin=[]  PParamMax=[]  IParamMin=[]  IParamMax=[]  DParamMin=[]  DParamMax=[]  NParamMin=[]  NParamMax=[]  KbParamMin=[]  KbParamMax=[]  KtParamMin=[]  KtParamMax=[]  POutMin=[]  POutMax=[]  IOutMin=[]  IOutMax=[]  DOutMin=[]  DOutMax=[]  NOutMin=[]  NOutMax=[]  KbOutMin=[]  KbOutMax=[]  KtOutMin=[]  KtOutMax=[]  IntegratorOutMin=[]  IntegratorOutMax=[]  FilterOutMin=[]  FilterOutMax=[]  SumOutMin=[]  SumOutMax=[]  SumI1OutMin=[]  SumI1OutMax=[]  SumI2OutMin=[]  SumI2OutMax=[]  SumI3OutMin=[]  SumI3OutMax=[]  SumDOutMin=[]  SumDOutMax=[]  SaturationOutMin=[]  SaturationOutMax=[]  IntegratorContinuousStateAttributes=''  IntegratorStateMustResolveToSignalObject=off  IntegratorRTWStateStorageClass=Auto  FilterContinuousStateAttributes=''  FilterStateMustResolveToSignalObject=off  FilterRTWStateStorageClass=Auto
  Sum1 : Sum  Inputs=|+-  OutDataType=fixdt(1, 16)  OutScaling=2^0
  Sum16 : Sum  Inputs=|+-  OutDataType=fixdt(1, 16)  OutScaling=2^0
  Sum2 : Sum  Inputs=|+-  OutDataType=fixdt(1, 16)  OutScaling=2^0
  m_theta : Outport  OutDataType=fixdt(1, 16)  OutScaling=2^0
  m_phi : Outport  Port=2  OutDataType=fixdt(1, 16)  OutScaling=2^0
  m_psi : Outport  Port=3  OutDataType=fixdt(1, 16)  OutScaling=2^0
  wires:
  Gain6/1 -> Sum16/2
  Sum16/1 -> PID rTheta OPT/1  "e_theta_hm"
  theta_hm_set/1 -> Sum16/1
  Sum2/1 -> PID rPhi OPT/1  "e_phi_hm"
  PID rPhi OPT/1 -> m_phi/1
  Gain1/1 -> Sum2/2
  vx_opt/1 -> Gain6/1
  PID rTheta OPT/1 -> m_theta/1
  phi_hm_set/1 -> Sum2/1
  rpsi_hm_set/1 -> Sum1/1
  PID rPsi OPT/1 -> Gain/1
  vy_opt/1 -> Gain1/1
  Sum1/1 -> PID rPsi OPT/1
  rpsi_opt/1 -> Sum1/2
  Gain/1 -> m_psi/1

== system System_Design_Quadrocopter/Quadrocopter/Dynamics/Equation of Motion Translation pos-vel-acc B-Frame/Equation of Motion Translation vel B-Frame ==
  vxe : Inport  OutDataType=fixdt(1, 16)  OutScaling=2^0
  vye : Inport  Port=2  OutDataType=fixdt(1, 16)  OutScaling=2^0
  vze : Inport  Port=3  OutDataType=fixdt(1, 16)  OutScaling=2^0
  phi : Inport  Port=4  OutDataType=fixdt(1, 16)  OutScaling=2^0
  theta : Inport  Port=5  OutDataType=fixdt(1, 16)  OutScaling=2^0
  psi : Inport  Port=6  OutDataType=fixdt(1, 16)  OutScaling=2^0
  Rotation matrix : Stateflow chart  AncestorBlock=Copter_Library/Quadrocopter model/Rotation matrix  TreatAsAtomicUnit=on
  u : Outport  OutDataType=fixdt(1, 16)  OutScaling=2^0
  v : Outport  Port=2  OutDataType=fixdt(1, 16)  OutScaling=2^0
  w : Outport  Port=3  OutDataType=fixdt(1, 16)  OutScaling=2^0
  wires:
  phi/1 -> Rotation matrix/1(phi)
  theta/1 -> Rotation matrix/2(theta)
  psi/1 -> Rotation matrix/3(psi)
  Rotation matrix/2(v) -> v/1
  vxe/1 -> Rotation matrix/4(vxe)
  vye/1 -> Rotation matrix/5(vye)
  vze/1 -> Rotation matrix/6(vze)
  Rotation matrix/1(u) -> u/1
  Rotation matrix/3(w) -> w/1

== system System_Design_Quadrocopter/Quadrocopter/Remote Control/Square_path_stimuli/Signal Builder ==
  Demux : Demux  Tag=STV Demux
  FromWs : FromWorkspace  Tag=STV FromWs  VariableName=tuvar  SampleTime=0  SigBuilderData=DataTag30  VnvData=DataTag31
      SigBuilderData=|
      | common.afterFinalStr = 'Extrapolate'
      | common.sampleTime = 0
      | dataSet.timeRange = [0 35]
      | dataSet.name = 'Group 1'
      | sbobj.Groups.Name = 'Group 1'
      | sbobj.Groups.Signals(1).Name = 'Signal 1'
      | sbobj.Groups.Signals(1).XData = [0 6 6 8 8 35]
      | sbobj.Groups.Signals(1).YData = [0 0 1 1 0 0]
      | sbobj.Groups.Signals(2).Name = 'Signal 2'
      | sbobj.Groups.Signals(2).XData = [0 15 15 17 17 35]
      | sbobj.Groups.Signals(2).YData = [0 0 1 1 0 0]
      | sbobj.Groups.Signals(3).Name = 'Signal 3'
      | sbobj.Groups.Signals(3).XData = [0 22 22 24 24 35]
      | sbobj.Groups.Signals(3).YData = [0 0 1 1 0 0]
      | sbobj.Groups.Signals(4).Name = 'Signal 4'
      | sbobj.Groups.Signals(4).XData = [0 30 30 32 32 35]
      | sbobj.Groups.Signals(4).YData = [0 0 1 1 0 0]
  Signal 1 : Outport  Tag=STV Outport  OutDataType=fixdt(1, 16)  OutScaling=2^0
  Signal 2 : Outport  Tag=STV Outport  Port=2
  Signal 3 : Outport  Tag=STV Outport  Port=3
  Signal 4 : Outport  Tag=STV Outport  Port=4
  wires:
  Demux/1 -> Signal 1/1
  FromWs/1 -> Demux/1
  Demux/2 -> Signal 2/1
  Demux/3 -> Signal 3/1
  Demux/4 -> Signal 4/1

== system System_Design_Quadrocopter/Quadrocopter/Remote Control/Square_path_stimuli/Subsystem1 ==
  In1 : Inport
  Gain1 : Gain  Gain=Gain_  ParameterDataType=fixdt(1, 16)  ParameterScaling=2^0  OutDataType=fixdt(1, 16)  OutScaling=2^0
  Out1 : Outport
  wires:
  Gain1/1 -> Out1/1
  In1/1 -> Gain1/1

== system System_Design_Quadrocopter/Quadrocopter/Remote Control/Square_path_stimuli/Subsystem2 ==
  In1 : Inport
  Gain1 : Gain  Gain=Gain_  ParameterDataType=fixdt(1, 16)  ParameterScaling=2^0  OutDataType=fixdt(1, 16)  OutScaling=2^0
  Out1 : Outport
  wires:
  Gain1/1 -> Out1/1
  In1/1 -> Gain1/1

== system System_Design_Quadrocopter/Quadrocopter/Remote Control/Square_path_stimuli/Subsystem3 ==
  In1 : Inport
  Gain1 : Gain  Gain=Gain_  ParameterDataType=fixdt(1, 16)  ParameterScaling=2^0  OutDataType=fixdt(1, 16)  OutScaling=2^0
  Out1 : Outport
  wires:
  Gain1/1 -> Out1/1
  In1/1 -> Gain1/1

== system System_Design_Quadrocopter/Quadrocopter/Remote Control/Square_path_stimuli/Subsystem4 ==
  In1 : Inport
  Gain1 : Gain  Gain=Gain_  ParameterDataType=fixdt(1, 16)  ParameterScaling=2^0  OutDataType=fixdt(1, 16)  OutScaling=2^0
  Out1 : Outport
  wires:
  Gain1/1 -> Out1/1
  In1/1 -> Gain1/1

== system System_Design_Quadrocopter/Quadrocopter/Sensors/Optical System/Rotation rpsi ==
  IdealSig : Inport  OutDataType=fixdt(1, 16)  OutScaling=2^0
  Add : Sum  OutDataType=fixdt(1, 16)  OutScaling=2^-10
  Constant : Constant  Value=Opt_Ori_SG  OutDataType=fixdt(1, 16)  OutScaling=2^0
  Dead Zone : DeadZone  LowerValue=0  UpperValue=0  SaturateOnIntegerOverflow=on
  Embedded MATLAB Function : Stateflow chart  TreatAsAtomicUnit=on
  Product1 : Product  OutDataType=fixdt(1, 16)  OutScaling=2^0  RndMeth=Zero
  Random Number : RandomNumber  Variance=Opt_Var  Seed=234234  SampleTime=Opt_Var_ST
  Saturation : Saturate  UpperLimit=Opt_Limit  LowerLimit=-Opt_Limit  OutDataType=fixdt(1, 16)  OutScaling=2^0
  Switched transport delay for linearization : TransportDelay  DelayTime=Opt_Delay  PadeOrder=2
  Zero-Order Hold2 : ZeroOrderHold  SampleTime=Opt_ST
  OptSig : Outport  OutDataType=fixdt(1, 16)  OutScaling=2^0
  wires:
  Add/1 -> Embedded MATLAB Function/1(Sig), Dead Zone/1
  Embedded MATLAB Function/1(Fac) -> Product1/2
  Product1/1 -> Add/1
  Saturation/1 -> Zero-Order Hold2/1
  Dead Zone/1 -> Saturation/1
  Zero-Order Hold2/1 -> Switched transport delay for linearization/1
  Random Number/1 -> Product1/1
  Switched transport delay for linearization/1 -> OptSig/1
  IdealSig/1 -> Add/2
  Constant/1 -> Embedded MATLAB Function/2(Gain)

== system System_Design_Quadrocopter/Quadrocopter/Sensors/Optical System/Translation VX ==
  IdealSig : Inport  OutDataType=fixdt(1, 16)  OutScaling=2^0
  Add : Sum  OutDataType=fixdt(1, 16)  OutScaling=2^-10
  Constant : Constant  Value=Opt_Ori_SG  OutDataType=fixdt(1, 16)  OutScaling=2^0
  Dead Zone : DeadZone  LowerValue=0  UpperValue=0  SaturateOnIntegerOverflow=on
  Embedded MATLAB Function : Stateflow chart  TreatAsAtomicUnit=on
  Product1 : Product  OutDataType=fixdt(1, 16)  OutScaling=2^0  RndMeth=Zero
  Random Number : RandomNumber  Variance=Opt_Var  Seed=234234  SampleTime=Opt_Var_ST
  Saturation : Saturate  UpperLimit=Opt_Limit  LowerLimit=-Opt_Limit  OutDataType=fixdt(1, 16)  OutScaling=2^0
  Switched transport delay for linearization : TransportDelay  DelayTime=Opt_Delay  PadeOrder=2
  Zero-Order Hold2 : ZeroOrderHold  SampleTime=Opt_ST
  OptSig : Outport  OutDataType=fixdt(1, 16)  OutScaling=2^0
  wires:
  Add/1 -> Embedded MATLAB Function/1(Sig), Dead Zone/1
  Embedded MATLAB Function/1(Fac) -> Product1/2
  Product1/1 -> Add/1
  Saturation/1 -> Zero-Order Hold2/1
  Dead Zone/1 -> Saturation/1
  Zero-Order Hold2/1 -> Switched transport delay for linearization/1
  Random Number/1 -> Product1/1
  Switched transport delay for linearization/1 -> OptSig/1
  IdealSig/1 -> Add/2
  Constant/1 -> Embedded MATLAB Function/2(Gain)

== system System_Design_Quadrocopter/Quadrocopter/Sensors/Optical System/Translation VY ==
  IdealSig : Inport  OutDataType=fixdt(1, 16)  OutScaling=2^0
  Add : Sum  OutDataType=fixdt(1, 16)  OutScaling=2^-10
  Constant : Constant  Value=Opt_Ori_SG  OutDataType=fixdt(1, 16)  OutScaling=2^0
  Dead Zone : DeadZone  LowerValue=0  UpperValue=0  SaturateOnIntegerOverflow=on
  Embedded MATLAB Function : Stateflow chart  TreatAsAtomicUnit=on
  Product1 : Product  OutDataType=fixdt(1, 16)  OutScaling=2^0  RndMeth=Zero
  Random Number : RandomNumber  Variance=Opt_Var  Seed=234234  SampleTime=Opt_Var_ST
  Saturation : Saturate  UpperLimit=Opt_Limit  LowerLimit=-Opt_Limit  OutDataType=fixdt(1, 16)  OutScaling=2^0
  Switched transport delay for linearization : TransportDelay  DelayTime=Opt_Delay  PadeOrder=2
  Zero-Order Hold2 : ZeroOrderHold  SampleTime=Opt_ST
  OptSig : Outport  OutDataType=fixdt(1, 16)  OutScaling=2^0
  wires:
  Add/1 -> Embedded MATLAB Function/1(Sig), Dead Zone/1
  Embedded MATLAB Function/1(Fac) -> Product1/2
  Product1/1 -> Add/1
  Saturation/1 -> Zero-Order Hold2/1
  Dead Zone/1 -> Saturation/1
  Zero-Order Hold2/1 -> Switched transport delay for linearization/1
  Random Number/1 -> Product1/1
  Switched transport delay for linearization/1 -> OptSig/1
  IdealSig/1 -> Add/2
  Constant/1 -> Embedded MATLAB Function/2(Gain)

== system System_Design_Quadrocopter/Quadrocopter/Sensors/acc_ax_sensor/Sensor Noise ==
  Enable : EnablePort  PropagateVarSize=During execution
  Random Number3 : RandomNumber  Variance=0.0003  Seed=676  SampleTime=Ts
  Noise : Outport
  wires:
  Random Number3/1 -> Noise/1

== system System_Design_Quadrocopter/Quadrocopter/Sensors/acc_ay_sensor/Sensor Noise ==
  Enable : EnablePort  PropagateVarSize=During execution
  Random Number2 : RandomNumber  Variance=0.0003  Seed=4564  SampleTime=0.01
  Noise : Outport
  wires:
  Random Number2/1 -> Noise/1

== system System_Design_Quadrocopter/Quadrocopter/Sensors/rate_phi_sensor/Sensor Noise ==
  Enable : EnablePort  PropagateVarSize=During execution
  Random Number1 : RandomNumber  Variance=3.0462e-8  Seed=45632  SampleTime=0.01
  Noise : Outport
  wires:
  Random Number1/1 -> Noise/1

== system System_Design_Quadrocopter/Quadrocopter/Sensors/rate_psi_sensor/Sensor Noise ==
  Enable : EnablePort  PropagateVarSize=During execution
  Random Number4 : RandomNumber  Variance=3.0462e-8  Seed=1634  SampleTime=0.01
  Noise : Outport
  wires:
  Random Number4/1 -> Noise/1

== system System_Design_Quadrocopter/Quadrocopter/Sensors/rate_theta_sensor/Sensor Noise ==
  Enable : EnablePort  PropagateVarSize=During execution
  Random Number5 : RandomNumber  Variance=3.0462e-8  Seed=4731  SampleTime=0.01
  Noise : Outport
  wires:
  Random Number5/1 -> Noise/1

== matlab function Quadrocopter/Control/Embedded PID Control ==
  settings: updateMethod=DISCRETE  sampleTime=0.005
  data: u input double; y output double
function y = fcn(u)
%#eml
persistent e_r_Roll_1 e_Roll_1 r_Roll_I_State r_Roll_Filter_State 
persistent e_r_Pitch_1 e_Pitch_1 r_Pitch_I_State r_Pitch_Filter_State 
persistent e_r_Yaw_1 r_Yaw_I_State r_Yaw_Filter_State
persistent M1_limited M2_limited M3_limited M4_limited 
%  first time initialization
if isempty(M1_limited) 
    M1_limited=uint8(0);
    M2_limited=uint8(0);
    M3_limited=uint8(0);
    M4_limited=uint8(0);
    e_r_Roll_1 = double(0);
    e_Roll_1 = double(0);
    r_Roll_I_State = double(0);
    r_Roll_Filter_State = double(0); 
    e_r_Pitch_1 = double(0);
    e_Pitch_1 = double(0);
    r_Pitch_I_State = double(0); 
    r_Pitch_Filter_State = double(0); 
    e_r_Yaw_1 = double(0); 
    r_Yaw_I_State = double(0); 
    r_Yaw_Filter_State = double(0);
end
IRoll = double(0);
FiltRoll = double(0);
IPitch = double(0);
FiltPitch = double(0);
Ts = 0.005; % sec
G = 9.810; % m/sec²
maxRemotePitch = 128;
maxRemoteRoll = 128;
maxRemoteYaw = 128;
maxPitchAngle = pi/4;
maxRollAngle  = pi/4;
maxYawRate = 200;
sensorSensitivityX = 340;
sensorSensitivityY = 340;
sensorSensitivityZ = 340;
copterState.gyroPOffset = 505;
copterState.gyroROffset = 505;
copterState.gyroYOffset = 505;
copterState.YawRateI_State = 0;
copterState.YawRateD_Filter = 0;
copterState.PitchRateI_State = 0;
copterState.PitchRateD_Filter = 0;
copterState.RollRateI_State = 0;
copterState.RollRateD_Filter = 0;
% copy inputs to variables with easy to know names
copterState.angVelRRaw =  u(3);
copterState.accYRaw = u(2);
copterState.angVelPRaw = u(4);
copterState.accXRaw = u(1);
copterState.accZRaw = 0; %not available
copterState.angVelYRaw = u(5);
copterState.remoteForceRaw = u(9);
copterState.remotePitchRaw = u(7);
copterState.remoteRollRaw = u(6);
copterState.remoteYawRaw = u(8);
copterState.accY = int16(0);
copterState.accX = int16(0);
copterState.accZ = int16(0);
copterState.angP = int16(0);
copterState.angR = int16(0);
copterState.angVelP = int16(0);
copterState.angVelR = int16(0);
copterState.angVelY = int16(0);
copterState.remotePitch = int16(0);
copterState.remoteRoll = int16(0);
copterState.remoteForce = int16(0);
copterState.remoteYaw = int16(0);
angP = double(0);
angR = double(0);

% Convert Data like in the copter
% Accelerometer
%%%%%%%%%%%%%%%%%
  %/* calculate the physical acceleration values in [(10 * m)/(s^2)], as needed by the control algorithm */
  copterState.accY = int16(((int32(copterState.accYRaw) * G) / sensorSensitivityY) / 10);
  copterState.accX = -int16(((int32(copterState.accXRaw) * G) / sensorSensitivityX) / 10);
  copterState.accZ = -int16(((int32(copterState.accZRaw) * G) / sensorSensitivityZ) / 10);
  %// [ 10000*rad ]
  copterState.angP = -int16(int32(copterState.accXRaw)*1000/340);
  copterState.angR = -int16(int32(copterState.accYRaw)*1000/340);
  
  % Gyroscopes [100 * rad/sec]
  %%%%%%%%%%%%%%
   copterState.angVelP     = -int16(double(copterState.angVelPRaw-copterState.gyroPOffset) * 0.938349);
   copterState.angVelR     = int16(double(copterState.angVelRRaw-copterState.gyroROffset) * 0.938349);
   copterState.angVelY     = -int16(double(copterState.angVelYRaw-copterState.gyroYOffset) * 0.938349);
   
   % Remote
   %%%%%%%%%%%%%
  copterState.remotePitch    = int16(maxPitchAngle*int32(copterState.remotePitchRaw-128)/maxRemotePitch);
  copterState.remoteRoll     = -int16(maxRollAngle*int32(copterState.remoteRollRaw-128)/maxRemoteRoll);
  copterState.remoteForce    = int16(copterState.remoteForceRaw); 
  copterState.remoteYaw      = int16(maxYawRate*int32(copterState.remoteYawRaw-128)/maxRemoteYaw);

% Set outputs to Values calculated last sample time
y = double([M1_limited;M2_limited;M3_limited;M4_limited]);
   
   angP = double(copterState.angP)/1000;
   angR = double(copterState.angR)/1000;
   
% calculate error values for the controlled angles
   % Pitch error 
   e_Pitch = double(copterState.remotePitch) - angP;
   % Roll error
   e_Roll = double(copterState.remoteRoll) - angR;
   % calculate controller output for the angles (I State & FilterState are not necessary cause only p is used
   [m_Roll, IRoll, FiltRoll] = PID(150,0.5,0,0,e_Roll,e_Roll_1,IRoll, FiltRoll, Ts);
   [m_Pitch, IPitch, FiltPitch] = PID(150,0.5,0,0,e_Pitch,e_Pitch_1,IPitch,FiltPitch,Ts);
      
   % Yaw Rate error
   e_r_Yaw = double(copterState.remoteYaw) - double(copterState.angVelY);
   % Pitch Rate error
   e_r_Pitch = m_Pitch - double(copterState.angVelP);
   % Roll Rate error
   e_r_Roll = m_Roll - double(copterState.angVelR);
   % calculate  controller output for rates
   [m_r_Yaw,r_Yaw_I_State, r_Yaw_Filter_State] = PID (70, ...
       0.5, 0,0,e_r_Yaw, e_r_Yaw_1, r_Yaw_I_State, r_Yaw_Filter_State,Ts);
   [m_r_Roll,r_Roll_I_State, r_Roll_Filter_State] = PID (70, ...
       0.5, 0,0,e_r_Roll, e_r_Roll_1, r_Roll_I_State, r_Roll_Filter_State,Ts);
   [m_r_Pitch,r_Pitch_I_State, r_Pitch_Filter_State] = PID (70, ...
       0.5, 0,0,e_r_Pitch, e_r_Pitch_1, r_Pitch_I_State, r_Pitch_Filter_State,Ts);
   
   % save error for next sample time
   e_Roll_1 = e_Roll;
   e_Pitch_1 = e_Pitch;
   e_r_Roll_1 = e_r_Roll;
   e_r_Pitch_1 = e_r_Pitch;
   e_r_Yaw_1 = e_r_Yaw;
 
   %//Calculate new setpoints of all motors
    M1 = (copterState.remoteForce-m_r_Pitch+m_r_Yaw);
    M2 = (copterState.remoteForce+m_r_Roll-m_r_Yaw);
    M3 = (copterState.remoteForce+m_r_Pitch+m_r_Yaw);
    M4 = (copterState.remoteForce-m_r_Roll-m_r_Yaw);
   
   
    %// saturate setpoint of motor1 to 0 if less and 255 if above
    if M1 < 0
      M1_limited = uint8(0);
    else
        if M1 > 255
            M1_limited = uint8(255); 
        else
            M1_limited=uint8(M1);
        end
    end
    
    %// saturate setpoint of motor2 to 0 if less and 255 if above
    if M2 < 0
      M2_limited = uint8(0);
    else
        if M2 > 255
          M2_limited = uint8(255); 
        else
          M2_limited=uint8(M2);
        end
    end

    %// saturate setpoint of motor3 to 0 if less and 255 if above
  if M3 < 0
      M3_limited = uint8(0);
  else
      if M3 > 255
        M3_limited = uint8(255); 
      else
         M3_limited=uint8(M3);
      end
  end
    
    %// saturate setpoint of motor4 to 0 if less and 255 if above
    if M4 < 0
      M4_limited = uint8(0);
    else
        if M4 > 255
           M4_limited = uint8(255); 
        else
           M4_limited=uint8(M4);
        end
    end

% This function calculates the next Value of the ?ideal? PID controller
function [ret, I_State, Filt_State] = PID (P, I, D, N, ek, ek_1, I_State, Filt_State, Ts)

if P ~= 0 
    if I ~= 0
        % calculate new itegral value
        I_State = ek * Ts * I + I_State;
    else
        I_State = 0;
    end

    if D ~= 0
        % calculate new derivative Value
        yd = (ek - ek_1)/Ts * D;

        % Filter the derivative  Value
        Filt_State = Ts * (yd -N*Filt_State)+ Filt_State ;
    else
        Filt_State = 0;
    end

    % Add all values and multiply P gain to all
    ret = (P * ek + I_State + Filt_State);

else
    ret = 0;
end


function ret16 = mult_fp (A, B, factor)
    ret32 = int32(A) * int32(B)/factor;
    if ret32 > 2^15-1
        ret16 = int16(2^15-1);
    else
        if ret32 < -2^15+1
            ret16 = int16(-2^15+1);
        else
            ret16 = int16(ret32);
        end
    end
% end of mult_fp    

function ret16 = div_fp(A, B, factor)
if B == 0
    display('divide by ZERO !!!!')
    ret16 = 2^16-1;
else
    ret32 = int32(A)*factor/int32(B);
     if ret32 > 2^15-1
        ret16 = int16(2^15-1);
    else
        if ret32 < -2^15+1
            ret16 = int16(-2^15+1);
        else
            ret16 = int16(ret32);
        end
    end
end
% end of div_fp

== matlab function Quadrocopter/Dynamics/Equation of Motion Translation pos-vel-acc B-Frame/Equation of Motion Translation vel B-Frame/Rotation matrix ==
  data: phi input double; theta input double; psi input double; u output double; v output double; vxe input double; vye input double; vze input double; w output double
function [u, v, w]   = input(phi, theta, psi, vxe, vye, vze)
% Transformation of E-frame to B-Frame
% R1_1 = cos(psi)*cos(theta);
% R2_1 = sin(psi)*cos(theta);
% R3_1 = -sin(theta);
% R1_2 = -sin(psi)*cos(phi)+cos(psi)*sin(theta)*sin(phi);
% R2_2 = cos(psi)*cos(phi)+sin(psi)*sin(theta)*sin(phi);
% R3_2 = cos(theta)*sin(phi);
% R1_3 = sin(psi)*sin(phi)+cos(psi)*sin(theta)*cos(phi);
% R2_3 = -cos(psi)*sin(phi)+sin(psi)*sin(theta)*cos(phi);
% R3_3 = cos(theta)*cos(phi);
% 
% T1_1 = 1;
% T2_1 = 0;
% T3_1 = 0;
% T1_2 = sin(phi)*tan(theta);
% T2_2 = cos(phi);
% T3_2 = sin(phi)/cos(theta);
% T1_3 = cos(phi)*tan(theta);
% T2_3 = -sin(phi);
% T3_3 = cos(phi)*cos(theta);

RTheta_inv  = [ cos(psi)*cos(theta), cos(theta)*sin(psi), -sin(theta);...
            cos(psi)*sin(phi)*sin(theta) - cos(phi)*sin(psi), cos(phi)*cos(psi) + sin(phi)*sin(psi)*sin(theta), cos(theta)*sin(phi);...
            sin(phi)*sin(psi) + cos(phi)*cos(psi)*sin(theta), cos(phi)*sin(psi)*sin(theta) - cos(psi)*sin(phi), cos(phi)*cos(theta)];
VB=RTheta_inv*[vxe; vye; vze];
u=VB(1);
v=VB(2);
w=VB(3);
% RTheta =[cos(psi)*cos(theta), -sin(psi)*cos(phi)+cos(psi)*sin(theta)*sin(phi), sin(psi)*sin(phi)+cos(psi)*sin(theta)*cos(phi);...
%         sin(psi)*cos(theta),  cos(psi)*cos(phi)+sin(psi)*sin(theta)*sin(phi), -cos(psi)*sin(phi)+sin(psi)*sin(theta)*cos(phi);...
%         -sin(theta), cos(theta)*sin(phi), cos(theta)*cos(phi)];
% TTheta = [ 1, sin(phi)*tan(theta), cos(phi)*tan(theta);...
%            0, cos(phi), -sin(phi);...
%            0, sin(phi)/cos(theta), cos(phi)*cos(theta)];
